simulink model "SourceAndSink_Demo"  (R2017b)
settings: Solver=VariableStepAuto  StartTime=0.0  StopTime=10.0  RelTol=1e-3
libraries: simulink x1
settings Model: Creator=javed  LastModifiedBy=javed

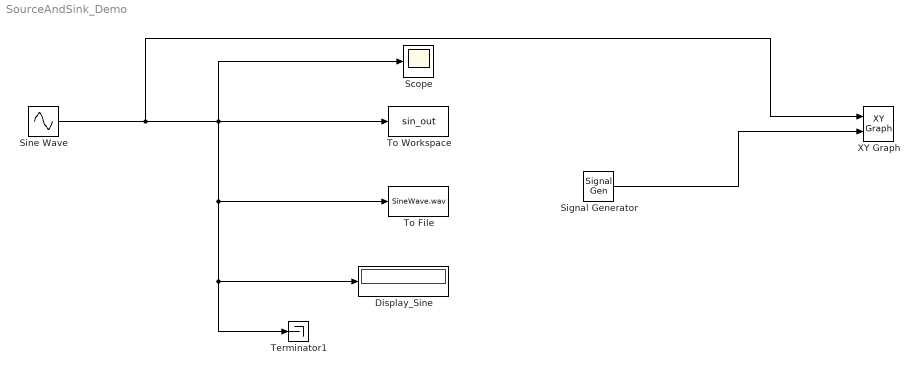
== system SourceAndSink_Demo ==
  Display_Sine : Display
  Scope : Scope
  Signal Generator : SignalGenerator  Units=rad/sec
  Sine Wave : Sin  Phase=pi/2  SampleTime=0
  Terminator1 : Terminator
  To File : ToFile  Filename=SineWave.wav  SaveFormat=Timeseries
  To Workspace : ToWorkspace  VariableName=sin_out  SaveFormat=Timeseries  SampleTime=-1
  XY Graph : simulink/Sinks/XY Graph  xmin=-1  xmax=1  ymin=-1  ymax=1  st=-1
  wires:
  Sine Wave/1 -> XY Graph/1, Scope/1, To File/1, Terminator1/1, Display_Sine/1, To Workspace/1
  Signal Generator/1 -> XY Graph/2
